simulink model "ModeManager_1"  (R2024a)
settings: Solver=VariableStepAuto  StartTime=0.0  StopTime=10.0  RelTol=1e-3
undefined symbols (not defined in the file or in its folder): canChannel
libraries: canlib x5, canmsglib x5
settings Model: DataDictionary=BMS_System_dict1.sldd  Creator=hirah  LastModifiedBy=hirah

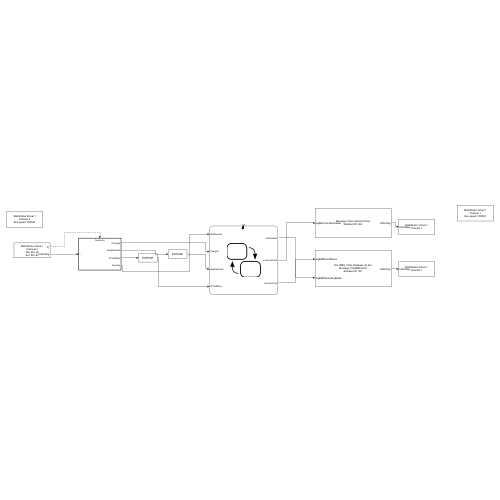
[thumbnail: Simulink's stored preview of the top-level diagram]
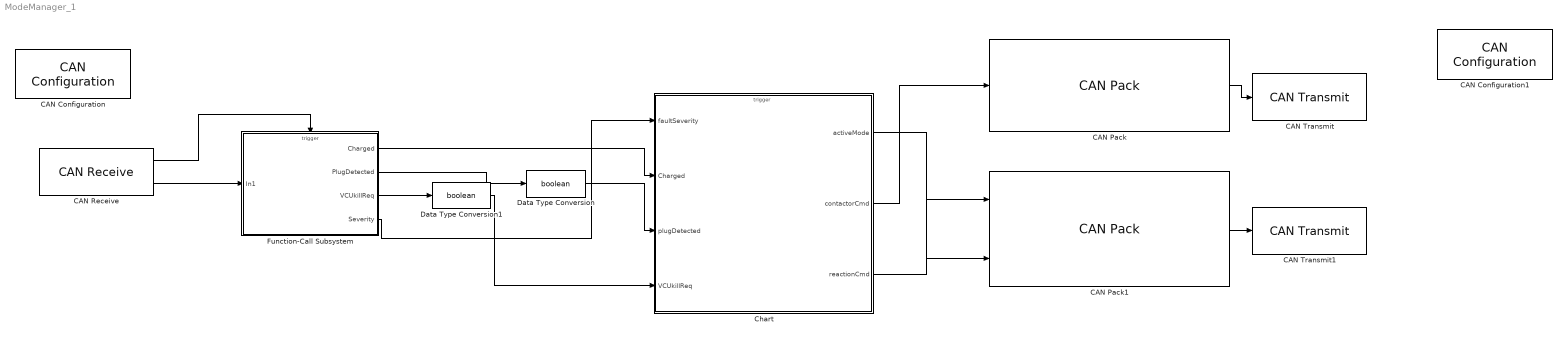
== system ModeManager_1 ==
  CAN Configuration : canlib/CAN Configuration  BlockHandle=570.0001  Device=MathWorks Virtual 1 (Channel 2)  DeviceMenu=MathWorks Virtual 1 (Channel 2)  ObjConstructor=canChannel('MathWorks', 'Virtual 1', 2)  BusSpeed=500000  EnableBitParameters=off  AckMode=Normal
  CAN Configuration1 : canlib/CAN Configuration  BlockHandle=570.0001  Device=MathWorks Virtual 1 (Channel 1)  DeviceMenu=MathWorks Virtual 1 (Channel 1)  ObjConstructor=canChannel('MathWorks', 'Virtual 1', 1)  BusSpeed=500000  EnableBitParameters=off  AckMode=Normal
  CAN Pack : canmsglib/CAN Pack  CANdbFile=C:\Users\hirah\Downloads\BMS_CAN_Database (5).dbc  MsgList=frmContactorControl  MsgName=frmContactorControl  MsgIDType=Standard (11-bit identifier)  MsgIdentifier=262  MsgLength=3  Remote=off  ApplyMinMax=off  BusOutput=off  SignalInfo={ 'sigMainContactorState', '8', '8', 'LE', 'unsigned', 'Standard', '0', '1', '0', '0', '3' }
      settings: LibrarySourceBlock=canlib/CAN Pack  DataFormat=manually specified signals
  CAN Pack1 : canmsglib/CAN Pack  CANdbFile=C:\Users\hirah\Downloads\BMS_CAN_Database (5).dbc  MsgList=frmBMStoVCU  MsgName=frmBMStoVCU  MsgIDType=Standard (11-bit identifier)  MsgIdentifier=321  MsgLength=2  Remote=off  ApplyMinMax=off  BusOutput=off  SignalInfo={'sigBMSFaultStatus','8','8','LE','unsigned','Standard','0','1','0','0','3';'sigBMSOperatingMode','0','8','LE','unsigned','Standard','0','1','0','0','5'}
      settings: LibrarySourceBlock=canlib/CAN Pack  DataFormat=CANdb specified signals
  CAN Receive : canlib/CAN Receive  BlockHandle=729.0002  Device=MathWorks Virtual 1 (Channel 2)  DeviceMenu=MathWorks Virtual 1 (Channel 2)  ObjConstructor=canChannel('MathWorks', 'Virtual 1', 2)  EnableStandardIDsFilter=off  StdIDsCombo=Allow all  StandardIDs=261  EnableExtendedIDsFilter=off  ExtIDsCombo=Allow all  ExtendedIDs=0  SampleTime=0.01  MsgsPerTimestep=all  InternalFilterUpdateStatus=on  BusOutput=off
  CAN Transmit : canlib/CAN Transmit  BlockHandle=714.0001  Device=MathWorks Virtual 1 (Channel 1)  DeviceMenu=MathWorks Virtual 1 (Channel 1)  ObjConstructor=canChannel('MathWorks', 'Virtual 1', 1)  EnableEventTransmit=off  EnablePeriodicTransmit=off  MessagePeriod=1.000
  CAN Transmit1 : canlib/CAN Transmit  BlockHandle=714.0001  Device=MathWorks Virtual 1 (Channel 1)  DeviceMenu=MathWorks Virtual 1 (Channel 1)  ObjConstructor=canChannel('MathWorks', 'Virtual 1', 1)  EnableEventTransmit=off  EnablePeriodicTransmit=off  MessagePeriod=1.000
  Chart : Stateflow chart  TreatAsAtomicUnit=on
  Data Type Conversion : DataTypeConversion  OutDataTypeStr=boolean  SaturateOnIntegerOverflow=off  RndMeth=Floor
  Data Type Conversion1 : DataTypeConversion  OutDataTypeStr=boolean  SaturateOnIntegerOverflow=off  RndMeth=Floor
  Function-Call Subsystem : Subsystem  TreatAsAtomicUnit=on
  wires:
  CAN Receive/2 -> Function-Call Subsystem/1(In1)
  CAN Receive/1 -> Function-Call Subsystem/Trigger
  Function-Call Subsystem/1(Charged) -> Chart/2(Charged)
  Function-Call Subsystem/2(PlugDetected) -> Data Type Conversion/1
  Function-Call Subsystem/3(VCUkillReq) -> Data Type Conversion1/1
  Function-Call Subsystem/4(Severity) -> Chart/1(faultSeverity)
  CAN Pack1/1 -> CAN Transmit1/1
  CAN Pack/1 -> CAN Transmit/1
  Chart/2(contactorCmd) -> CAN Pack/1
  Chart/1(activeMode) -> CAN Pack1/2
  Chart/3(reactionCmd) -> CAN Pack1/1
  Data Type Conversion/1 -> Chart/3(plugDetected)
  Data Type Conversion1/1 -> Chart/4(VCUkillReq)

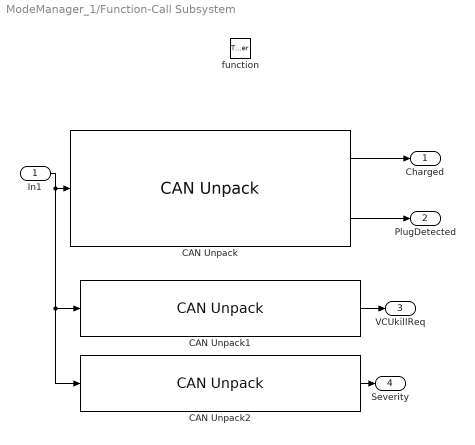
== system ModeManager_1/Function-Call Subsystem ==
  In1 : Inport
  function : TriggerPort  TriggerType=function-call  VariantControl=(inherit)
  CAN Unpack : canmsglib/CAN Unpack  CANdbFile=C:\Users\hirah\Downloads\BMS_CAN_Database (5).dbc  MsgList=frmChargingStatus  MsgName=frmChargingStatus  MsgIDType=Standard (11-bit identifier)  MsgIdentifier=266  MsgLength=3  SignalInfo={ 'sigChargeComplete', '16', '8', 'LE', 'unsigned', 'Standard', '0', '1', '0', '0', '1'; 'sigPlugStatus', '0', '8', 'LE', 'unsigned', 'Standard', '0', '1', '0', '0', '2' }  IDPort=off  TimestampPort=off  ErrorPort=off  RemotePort=off  LengthPort=off  StatusPort=off  ApplyMinMax=off
  CAN Unpack1 : canmsglib/CAN Unpack  CANdbFile=C:\Users\hirah\Downloads\BMS_CAN_Database (5).dbc  MsgList=frmVCUCommands  MsgName=frmVCUCommands  MsgIDType=Standard (11-bit identifier)  MsgIdentifier=320  MsgLength=3  SignalInfo={ 'sigVCUModeRequest', '0', '8', 'LE', 'unsigned', 'Standard', '0', '1', '0', '0', '5' }  IDPort=off  TimestampPort=off  ErrorPort=off  RemotePort=off  LengthPort=off  StatusPort=off  ApplyMinMax=off
  CAN Unpack2 : canmsglib/CAN Unpack  CANdbFile=C:\Users\hirah\Downloads\BMS_CAN_Database (5).dbc  MsgList=frmDiagnosticDTC  MsgName=frmDiagnosticDTC  MsgIDType=Standard (11-bit identifier)  MsgIdentifier=264  MsgLength=3  SignalInfo={ 'sigDTCSeverity1', '16', '8', 'LE', 'unsigned', 'Standard', '0', '1', '0', '0', '3' }  IDPort=off  TimestampPort=off  ErrorPort=off  RemotePort=off  LengthPort=off  StatusPort=off  ApplyMinMax=off
  Charged : Outport
  PlugDetected : Outport  Port=2
  VCUkillReq : Outport  Port=3
  Severity : Outport  Port=4
  wires:
  In1/1 -> CAN Unpack2/1, CAN Unpack1/1, CAN Unpack/1
  CAN Unpack/1 -> Charged/1
  CAN Unpack/2 -> PlugDetected/1
  CAN Unpack1/1 -> VCUkillReq/1
  CAN Unpack2/1 -> Severity/1

== stateflow chart ModeManager_1/Chart ==
  settings: executeAtInitialization=1  initializeOutput=1
  state INIT
    entry: activeMode = 0;
    contactorCmd = false;
    reactionCmd = 0;
  state CHARGING
    entry: activeMode = 2;
    contactorCmd = true;
    reactionCmd = 0;
  state NORMAL
    entry: activeMode = 1;
    contactorCmd = true;
    reactionCmd = 0;
  state SLEEP
    entry: activeMode = 5;
    contactorCmd = false;
    reactionCmd = 0;
  state LIMP
    entry: activeMode = 3;
    contactorCmd = true;
    reactionCmd = 1;
  state SAFE_STATE
    entry: activeMode = 4;
    contactorCmd = false;
    reactionCmd = 2;
  SLEEP -> INIT : [canNM_Wake == true || kl15_signal == true]
  (default) -> INIT
  SAFE_STATE -> INIT : [after(5, sec)]
  INIT -> NORMAL : [[after(0.5, sec)]]
  NORMAL -> CHARGING [order 1] : [plugDetected == 1]
  CHARGING -> NORMAL : [Charged == 1]
  NORMAL -> LIMP [order 2] : [faultSeverity == 1]
  NORMAL -> SAFE_STATE [order 3] : [faultSeverity == 2]
  NORMAL -> SLEEP [order 4] : [VCUkillReq == 1]
  LIMP -> SAFE_STATE : [faultSeverity == 2]
  data: faultSeverity input int32; Charged input; plugDetected input boolean; VCUkillReq input boolean; activeMode output int32 =0; contactorCmd output boolean =false; reactionCmd output int32 =0
  events: entry_ input RISING_EDGE_EVENT
